simulink model "IM_Controller_Design"  (R2024b)
settings: Solver=VariableStepAuto  StartTime=0.0  StopTime=10.0  RelTol=1e-3
undefined symbols (not defined in the file): Ci, ctrl, DiscIntNeverNeededParam, J, L_m, L_R, lamda_Rd_ref, p, PT1_flux, PT1_rotor, PT1_stator, T_Load, Ts, w_mech_ref
libraries: cstblocks x5
settings Model: Creator=overflow  LastModifiedBy=overflow

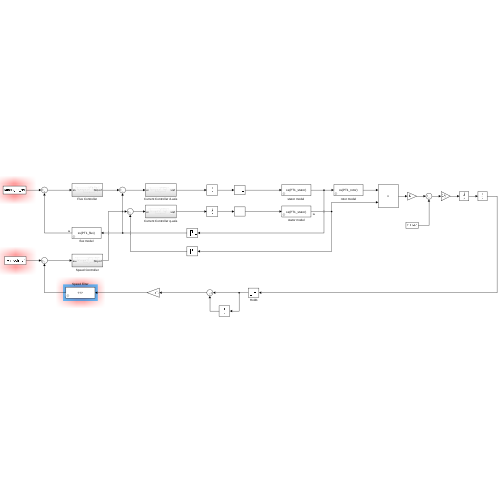
[thumbnail: Simulink's stored preview of the top-level diagram]
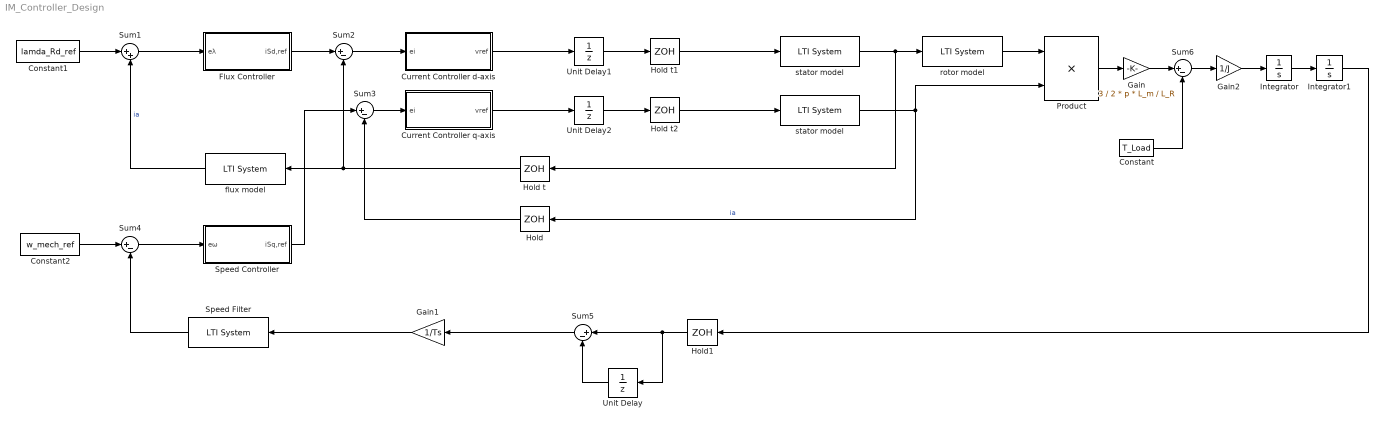
== system IM_Controller_Design ==
  " Hold" : ZeroOrderHold  SampleTime=-1
  " Hold t" : ZeroOrderHold  SampleTime=-1
  " Hold t1" : ZeroOrderHold  SampleTime=-1
  " Hold t2" : ZeroOrderHold  SampleTime=-1
  " Hold1" : ZeroOrderHold  SampleTime=-1
  Constant : Constant  Value=T_Load
  Constant1 : Constant  Value=lamda_Rd_ref
  Constant2 : Constant  Value=w_mech_ref
  Current Controller d-axis : Subsystem
  Current Controller q-axis : Subsystem
  Flux Controller : Subsystem
  Gain : Gain  Gain=3 / 2 * p * L_m / L_R
  Gain1 : Gain  Gain=1/Ts
  Gain2 : Gain  Gain=1/J
  Integrator : Integrator
  Integrator1 : Integrator
  Product : Product
  Speed Controller : Subsystem
  Speed Filter : cstblocks/LTI System  sys=Speed_Filter  IC=[]  PadeOrder=0
      link override Internal: InitialCondition=w_start
  Sum1 : Sum  Inputs=|++
  Sum{2..6} (5 alike) : Sum  Inputs=|+-
  Unit Delay : UnitDelay  SampleTime=-1  HasFrameUpgradeWarning=on
  Unit Delay1 : UnitDelay  SampleTime=-1  HasFrameUpgradeWarning=on
  Unit Delay2 : UnitDelay  SampleTime=-1  HasFrameUpgradeWarning=on
  flux model : cstblocks/LTI System  sys=ss(PT1_flux)  IC=[0]  PadeOrder=0
  rotor model : cstblocks/LTI System  sys=ss(PT1_rotor)  IC=[0]  PadeOrder=0
  stator model : cstblocks/LTI System  sys=ss(PT1_stator)  IC=[0]  PadeOrder=0
  "stator model " : cstblocks/LTI System  sys=ss(PT1_stator)  IC=[0]  PadeOrder=0
  wires:
  Sum1/1 -> Flux Controller/1(eλ)
  Flux Controller/1(iSd,ref) -> Sum2/1
  Sum2/1 -> Current Controller d-axis/1(ei)
  Sum3/1 -> Current Controller q-axis/1(ei)
  Speed Controller/1(iSq,ref) -> Sum3/1
  Sum4/1 -> Speed Controller/1(eω)
  flux model/1 -> Sum1/2  "ia"
  " Hold t"/1 -> Sum2/2, flux model/1
  Current Controller d-axis/1(vref) -> Unit Delay1/1
  " Hold t1"/1 -> "stator model "/1
  " Hold t2"/1 -> stator model/1
  Current Controller q-axis/1(vref) -> Unit Delay2/1
  " Hold"/1 -> Sum3/2
  "stator model "/1 -> " Hold t"/1, rotor model/1
  stator model/1 -> Product/2, " Hold"/1  "ia"
  Speed Filter/1 -> Sum4/2
  Unit Delay/1 -> Sum5/2
  " Hold1"/1 -> Unit Delay/1, Sum5/1
  Sum5/1 -> Gain1/1
  Integrator1/1 -> " Hold1"/1
  Constant/1 -> Sum6/2
  rotor model/1 -> Product/1
  Product/1 -> Gain/1
  Gain/1 -> Sum6/1
  Sum6/1 -> Gain2/1
  Integrator/1 -> Integrator1/1
  Gain2/1 -> Integrator/1
  Gain1/1 -> Speed Filter/1
  Unit Delay2/1 -> " Hold t2"/1
  Unit Delay1/1 -> " Hold t1"/1
  Constant1/1 -> Sum1/1
  Constant2/1 -> Sum4/1

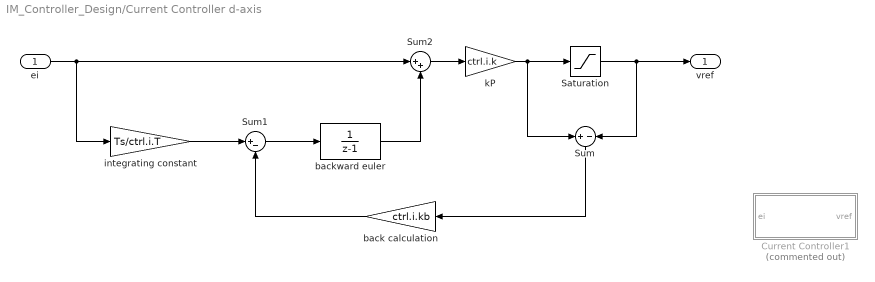
== system IM_Controller_Design/Current Controller d-axis ==
  ei : Inport
  Current Controller1 : Subsystem  Commented=on
  Saturation : Saturate  UpperLimit=ctrl.i.satP  LowerLimit=ctrl.i.satN
  Sum : Sum  Inputs=+|-
  Sum1 : Sum  Inputs=|+-
  Sum2 : Sum  Inputs=|++
  back calculation : Gain  Gain=ctrl.i.kb
  backward euler : DiscreteTransferFcn  Denominator=[1 -1]
  integrating constant : Gain  Gain=Ts/ctrl.i.T
  kP : Gain  Gain=ctrl.i.k
  vref : Outport
  wires:
  backward euler/1 -> Sum2/2
  kP/1 -> Saturation/1, Sum/1
  Sum2/1 -> kP/1
  ei/1 -> Sum2/1, integrating constant/1
  back calculation/1 -> Sum1/2
  Sum/1 -> back calculation/1
  Saturation/1 -> Sum/2, vref/1
  integrating constant/1 -> Sum1/1
  Sum1/1 -> backward euler/1

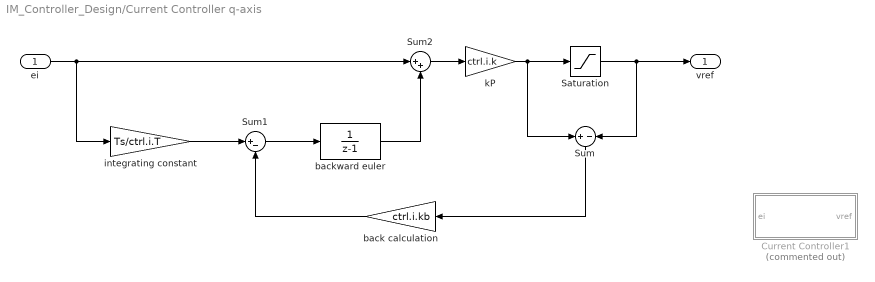
== system IM_Controller_Design/Current Controller q-axis ==
  ei : Inport
  Current Controller1 : Subsystem  Commented=on
  Saturation : Saturate  UpperLimit=ctrl.i.satP  LowerLimit=ctrl.i.satN
  Sum : Sum  Inputs=+|-
  Sum1 : Sum  Inputs=|+-
  Sum2 : Sum  Inputs=|++
  back calculation : Gain  Gain=ctrl.i.kb
  backward euler : DiscreteTransferFcn  Denominator=[1 -1]
  integrating constant : Gain  Gain=Ts/ctrl.i.T
  kP : Gain  Gain=ctrl.i.k
  vref : Outport
  wires:
  backward euler/1 -> Sum2/2
  kP/1 -> Saturation/1, Sum/1
  Sum2/1 -> kP/1
  ei/1 -> Sum2/1, integrating constant/1
  back calculation/1 -> Sum1/2
  Sum/1 -> back calculation/1
  Saturation/1 -> Sum/2, vref/1
  integrating constant/1 -> Sum1/1
  Sum1/1 -> backward euler/1

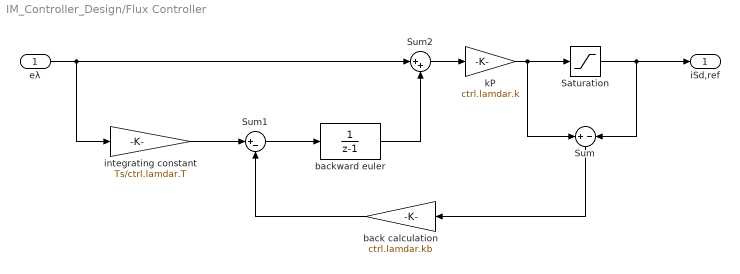
== system IM_Controller_Design/Flux Controller ==
  eλ : Inport
  Saturation : Saturate  UpperLimit=ctrl.lamdar.satP  LowerLimit=ctrl.lamdar.satN
  Sum : Sum  Inputs=+|-
  Sum1 : Sum  Inputs=|+-
  Sum2 : Sum  Inputs=|++
  back calculation : Gain  Gain=ctrl.lamdar.kb
  backward euler : DiscreteTransferFcn  Denominator=[1 -1]
  integrating constant : Gain  Gain=Ts/ctrl.lamdar.T
  kP : Gain  Gain=ctrl.lamdar.k
  iSd,ref : Outport
  wires:
  backward euler/1 -> Sum2/2
  kP/1 -> Saturation/1, Sum/1
  Sum2/1 -> kP/1
  eλ/1 -> Sum2/1, integrating constant/1
  back calculation/1 -> Sum1/2
  Sum/1 -> back calculation/1
  Saturation/1 -> Sum/2, iSd,ref/1
  integrating constant/1 -> Sum1/1
  Sum1/1 -> backward euler/1

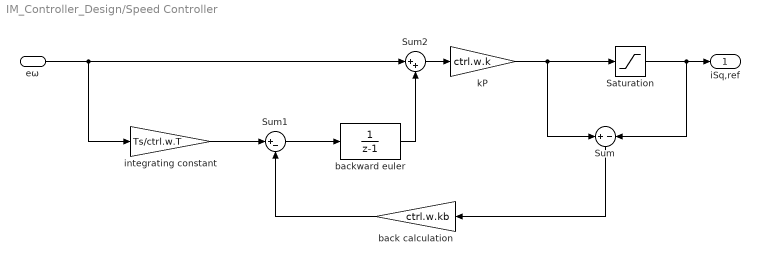
== system IM_Controller_Design/Speed Controller ==
  eω : Inport
  Saturation : Saturate  UpperLimit=ctrl.w.satP  LowerLimit=ctrl.w.satN
  Sum : Sum  Inputs=+|-
  Sum1 : Sum  Inputs=|+-
  Sum2 : Sum  Inputs=|++
  back calculation : Gain  Gain=ctrl.w.kb
  backward euler : DiscreteTransferFcn  Denominator=[1 -1]
  integrating constant : Gain  Gain=Ts/ctrl.w.T
  kP : Gain  Gain=ctrl.w.k
  iSq,ref : Outport
  wires:
  Sum1/1 -> backward euler/1
  Sum2/1 -> kP/1
  kP/1 -> Saturation/1, Sum/1
  Sum/1 -> back calculation/1
  integrating constant/1 -> Sum1/1
  back calculation/1 -> Sum1/2
  Saturation/1 -> Sum/2, iSq,ref/1
  backward euler/1 -> Sum2/2
  eω/1 -> integrating constant/1, Sum2/1

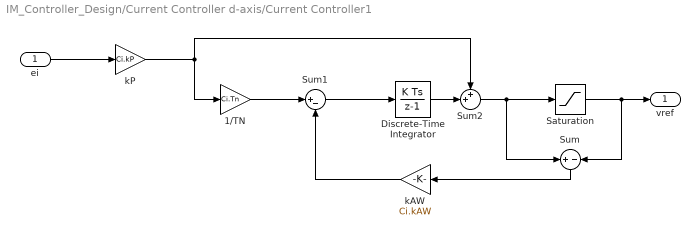
== system IM_Controller_Design/Current Controller d-axis/Current Controller1 ==
  ei : Inport
  1/TN : Gain  Gain=Ci.Tn
  Discrete-Time Integrator : DiscreteIntegrator  SampleTime=-1  ICPrevOutput=DiscIntNeverNeededParam  ICPrevScaledInput=DiscIntNeverNeededParam
  Saturation : Saturate
  Sum : Sum  Inputs=+|-
  Sum1 : Sum  Inputs=|+-
  Sum2 : Sum  Inputs=++|
  kAW : Gain  Gain=Ci.kAW
  kP : Gain  Gain=Ci.kP
  vref : Outport
  wires:
  kP/1 -> 1/TN/1, Sum2/1
  kAW/1 -> Sum1/2
  Sum/1 -> kAW/1
  Saturation/1 -> vref/1, Sum/2
  Sum2/1 -> Saturation/1, Sum/1
  ei/1 -> kP/1
  Discrete-Time Integrator/1 -> Sum2/2
  1/TN/1 -> Sum1/1
  Sum1/1 -> Discrete-Time Integrator/1

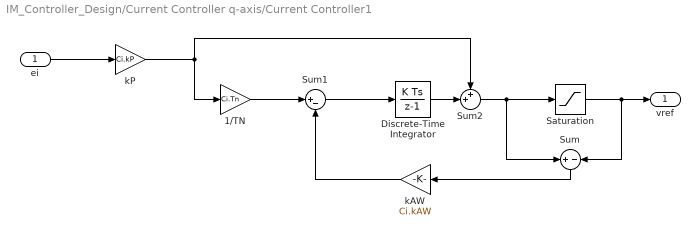
== system IM_Controller_Design/Current Controller q-axis/Current Controller1 ==
  ei : Inport
  1/TN : Gain  Gain=Ci.Tn
  Discrete-Time Integrator : DiscreteIntegrator  SampleTime=-1  ICPrevOutput=DiscIntNeverNeededParam  ICPrevScaledInput=DiscIntNeverNeededParam
  Saturation : Saturate
  Sum : Sum  Inputs=+|-
  Sum1 : Sum  Inputs=|+-
  Sum2 : Sum  Inputs=++|
  kAW : Gain  Gain=Ci.kAW
  kP : Gain  Gain=Ci.kP
  vref : Outport
  wires:
  kP/1 -> 1/TN/1, Sum2/1
  kAW/1 -> Sum1/2
  Sum/1 -> kAW/1
  Saturation/1 -> vref/1, Sum/2
  Sum2/1 -> Saturation/1, Sum/1
  ei/1 -> kP/1
  Discrete-Time Integrator/1 -> Sum2/2
  1/TN/1 -> Sum1/1
  Sum1/1 -> Discrete-Time Integrator/1
